simulink model "PREPROCESS"  (R2020b)
settings: Solver=FixedStepAuto  StartTime=0.0  StopTime=31622400  FixedStep=60  RelTol=1e-3
libraries: simulink x30
(part 2 of 2)

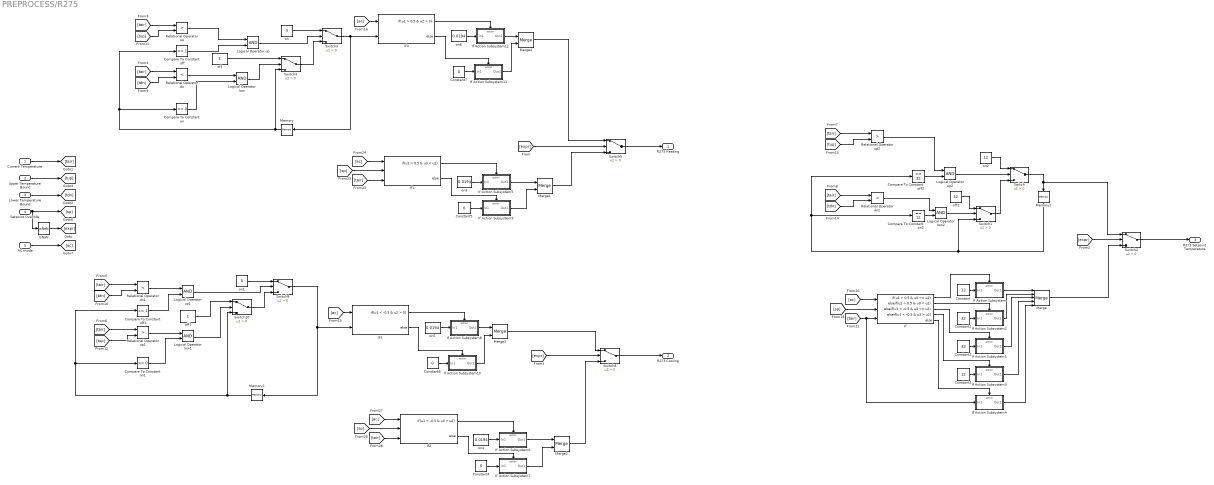
== system PREPROCESS/R275 ==
  Current Temperature : Inport
  Upper Temperature Bound : Inport  Port=2
  Lower Temperature Bound : Inport  Port=3
  Setpoint Override : Inport  Port=4
  AC mode : Inport  Port=5
  Compare To Constant off : simulink/Logic and Bit Operations/Compare To Constant  relop===  const=1  OutDataTypeStr=boolean
  Compare To Constant off1 : simulink/Logic and Bit Operations/Compare To Constant  relop===  const=1  OutDataTypeStr=boolean
  Compare To Constant off2 : simulink/Logic and Bit Operations/Compare To Constant  relop===  const=32  OutDataTypeStr=boolean
  Compare To Constant on : simulink/Logic and Bit Operations/Compare To Constant  relop===  const=0  OutDataTypeStr=boolean
  Compare To Constant on1 : simulink/Logic and Bit Operations/Compare To Constant  relop===  const=0  OutDataTypeStr=boolean
  Compare To Constant on2 : simulink/Logic and Bit Operations/Compare To Constant  relop===  const=12  OutDataTypeStr=boolean
  Constant : Constant  Value=12
  Constant1 : Constant  Value=32
  Constant2 : Constant  Value=32
  Constant3 : Constant  Value=12
  Constant{4..7} (4 alike) : Constant  Value=0
  If : If  NumInputs=3  IfExpression=u1 > 0.5 & u3 >= u2  ElseIfExpressions=u1 > 0.5 & u3 < u2, u1 < -0.5 & u3 <= u2, u1 < -0.5 & u3 > u2
  If Action Subsystem : Subsystem  TreatAsAtomicUnit=on
  If Action Subsystem1 : Subsystem  TreatAsAtomicUnit=on
  If Action Subsystem10 : Subsystem  TreatAsAtomicUnit=on
  If Action Subsystem11 : Subsystem  TreatAsAtomicUnit=on
  If Action Subsystem12 : Subsystem  TreatAsAtomicUnit=on
  If Action Subsystem2 : Subsystem  TreatAsAtomicUnit=on
  If Action Subsystem3 : Subsystem  TreatAsAtomicUnit=on
  If Action Subsystem4 : Subsystem  TreatAsAtomicUnit=on
  If Action Subsystem5 : Subsystem  TreatAsAtomicUnit=on
  If Action Subsystem6 : Subsystem  TreatAsAtomicUnit=on
  If Action Subsystem7 : Subsystem  TreatAsAtomicUnit=on
  If Action Subsystem8 : Subsystem  TreatAsAtomicUnit=on
  If Action Subsystem9 : Subsystem  TreatAsAtomicUnit=on
  If1 : If  NumInputs=3  IfExpression=u1 > 0.5 & u3 < u2
  If2 : If  NumInputs=3  IfExpression=u1 < -0.5 & u3 > u2
  If3 : If  NumInputs=2  IfExpression=u1 < -0.5 & u2 > 0
  If4 : If  NumInputs=2  IfExpression=u1 > 0.5 & u2 > 0
  IsNaN : RelationalOperator  Operator=isNaN  OutDataTypeStr=boolean  RndMeth=Simplest
  Logical Operator low : Logic  AllPortsSameDT=off  OutDataTypeStr=boolean
  Logical Operator low1 : Logic  AllPortsSameDT=off  OutDataTypeStr=boolean
  Logical Operator low2 : Logic  AllPortsSameDT=off  OutDataTypeStr=boolean
  Logical Operator up : Logic  AllPortsSameDT=off  OutDataTypeStr=boolean
  Logical Operator up1 : Logic  AllPortsSameDT=off  OutDataTypeStr=boolean
  Logical Operator up2 : Logic  AllPortsSameDT=off  OutDataTypeStr=boolean
  Memory : Memory
  Memory1 : Memory
  Memory2 : Memory  InitialCondition=12
  Merge : Merge  Inputs=5
  Merge{1..4} (4 alike) : Merge
  Relational Operator dn : RelationalOperator  Operator=<  OutDataTypeStr=boolean  RndMeth=Simplest
  Relational Operator dn1 : RelationalOperator  Operator=<  OutDataTypeStr=boolean  RndMeth=Simplest
  Relational Operator dn2 : RelationalOperator  Operator=<  OutDataTypeStr=boolean  RndMeth=Simplest
  Relational Operator up : RelationalOperator  Operator=>  OutDataTypeStr=boolean  RndMeth=Simplest
  Relational Operator up1 : RelationalOperator  Operator=>  OutDataTypeStr=boolean  RndMeth=Simplest
  Relational Operator up2 : RelationalOperator  Operator=>  OutDataTypeStr=boolean  RndMeth=Simplest
  Switch{,1..5,8..10} (9 alike) : Switch  Criteria=u2 > Threshold
  off : Constant
  off1 : Constant
  off2 : Constant  Value=32
  on : Constant  Value=0
  on1 : Constant  Value=0
  on2 : Constant  Value=12
  on{3..6} (4 alike) : Constant  Value=0.0194
  R273 Heating : Outport
  R273 Cooling : Outport  Port=2
  R273 Setpoint Temperature : Outport  Port=3
  wires:
  If3/1 -> If Action Subsystem8/Action
  If2/1 -> If Action Subsystem6/Action
  If Action Subsystem3/1(Out1) -> Merge/4
  [tair] -> If Action Subsystem4/1(In1), If/3
  [sp] -> If/2
  Relational Operator dn/1 -> Logical Operator low/1
  [tup] -> Relational Operator up/2
  Constant7/1 -> If Action Subsystem11/1(In1)
  [expr] -> Switch5/2
  If1/2 -> If Action Subsystem9/Action
  Merge2/1 -> Switch8/3
  on6/1 -> If Action Subsystem12/1(In1)
  If Action Subsystem10/1(Out1) -> Merge3/2
  [tair] -> If1/3
  on2/1 -> Switch/1
  IsNaN/1 -> [expr]
  If4/2 -> If Action Subsystem11/Action
  If Action Subsystem11/1(Out1) -> Merge4/2
  If4/1 -> If Action Subsystem12/Action
  Constant4/1 -> If Action Subsystem7/1(In1)
  Switch8/1 -> R273 Cooling/1
  [sp] -> If1/2
  If Action Subsystem8/1(Out1) -> Merge3/1
  on4/1 -> If Action Subsystem6/1(In1)
  If/5 -> If Action Subsystem4/Action
  [ac] -> If4/1
  Switch4/1 -> Switch3/3
  Switch9/1 -> If3/2, Memory1/1
  [sp] -> If2/2
  If3/2 -> If Action Subsystem10/Action
  Switch5/1 -> R273 Heating/1
  Constant6/1 -> If Action Subsystem10/1(In1)
  Relational Operator up2/1 -> Logical Operator up2/1
  on5/1 -> If Action Subsystem8/1(In1)
  Compare To Constant on/1 -> Logical Operator low/2
  Lower Temperature Bound/1 -> [tdn]
  Constant2/1 -> If Action Subsystem1/1(In1)
  If Action Subsystem4/1(Out1) -> Merge/5
  Compare To Constant off/1 -> Logical Operator up/2
  Merge4/1 -> Switch5/1
  If1/1 -> If Action Subsystem5/Action
  [ac] -> If3/1
  Merge3/1 -> Switch8/1
  AC mode/1 -> [ac]
  Logical Operator up/1 -> Switch3/2
  If Action Subsystem6/1(Out1) -> Merge2/1
  Memory/1 -> Compare To Constant on/1, Compare To Constant off/1, Switch4/3
  If/2 -> If Action Subsystem2/Action
  on3/1 -> If Action Subsystem5/1(In1)
  Merge1/1 -> Switch5/3
  If Action Subsystem9/1(Out1) -> Merge1/2
  If Action Subsystem/1(Out1) -> Merge/1
  Logical Operator low1/1 -> Switch10/2
  If/3 -> If Action Subsystem1/Action
  [tair] -> Relational Operator up2/1
  off1/1 -> Switch10/1
  [ac] -> If2/1
  Setpoint Override/1 -> IsNaN/1, [sp]
  Relational Operator dn2/1 -> Logical Operator low2/1
  If Action Subsystem12/1(Out1) -> Merge4/1
  Compare To Constant off2/1 -> Logical Operator up2/2
  Switch10/1 -> Switch9/3
  [ac] -> If/1
  Relational Operator up1/1 -> Logical Operator low1/1
  Relational Operator dn1/1 -> Logical Operator up1/1
  [tup] -> Relational Operator up1/2
  off/1 -> Switch4/1
  [expr] -> Switch2/2
  [expr] -> Switch8/2
  Constant/1 -> If Action Subsystem/1(In1)
  [tair] -> Relational Operator dn1/1
  [tair] -> Relational Operator up1/1
  [tdn] -> Relational Operator dn2/2
  Constant5/1 -> If Action Subsystem9/1(In1)
  If Action Subsystem7/1(Out1) -> Merge2/2
  Logical Operator low2/1 -> Switch1/2
  [tup] -> Relational Operator up2/2
  Merge/1 -> Switch2/3
  on/1 -> Switch3/1
  Constant3/1 -> If Action Subsystem3/1(In1)
  If/4 -> If Action Subsystem3/Action
  Logical Operator low/1 -> Switch4/2
  [tdn] -> Relational Operator dn1/2
  on1/1 -> Switch9/1
  Logical Operator up1/1 -> Switch9/2
  Compare To Constant off1/1 -> Logical Operator up1/2
  Relational Operator up/1 -> Logical Operator up/1
  Logical Operator up2/1 -> Switch/2
  Current Temperature/1 -> [tair]
  [tair] -> Relational Operator up/1
  [tair] -> Relational Operator dn/1
  If Action Subsystem1/1(Out1) -> Merge/3
  Compare To Constant on2/1 -> Logical Operator low2/2
  [tair] -> If2/3
  Switch3/1 -> Memory/1, If4/2
  Switch/1 -> Switch2/1, Memory2/1
  Constant1/1 -> If Action Subsystem2/1(In1)
  If Action Subsystem5/1(Out1) -> Merge1/1
  [tdn] -> Relational Operator dn/2
  Switch1/1 -> Switch/3
  off2/1 -> Switch1/1
  Memory1/1 -> Compare To Constant on1/1, Compare To Constant off1/1, Switch10/3
  Memory2/1 -> Compare To Constant on2/1, Compare To Constant off2/1, Switch1/3
  Upper Temperature Bound/1 -> [tup]
  Compare To Constant on1/1 -> Logical Operator low1/2
  [tair] -> Relational Operator dn2/1
  If/1 -> If Action Subsystem/Action
  [ac] -> If1/1
  If Action Subsystem2/1(Out1) -> Merge/2
  If2/2 -> If Action Subsystem7/Action
  Switch2/1 -> R273 Setpoint Temperature/1

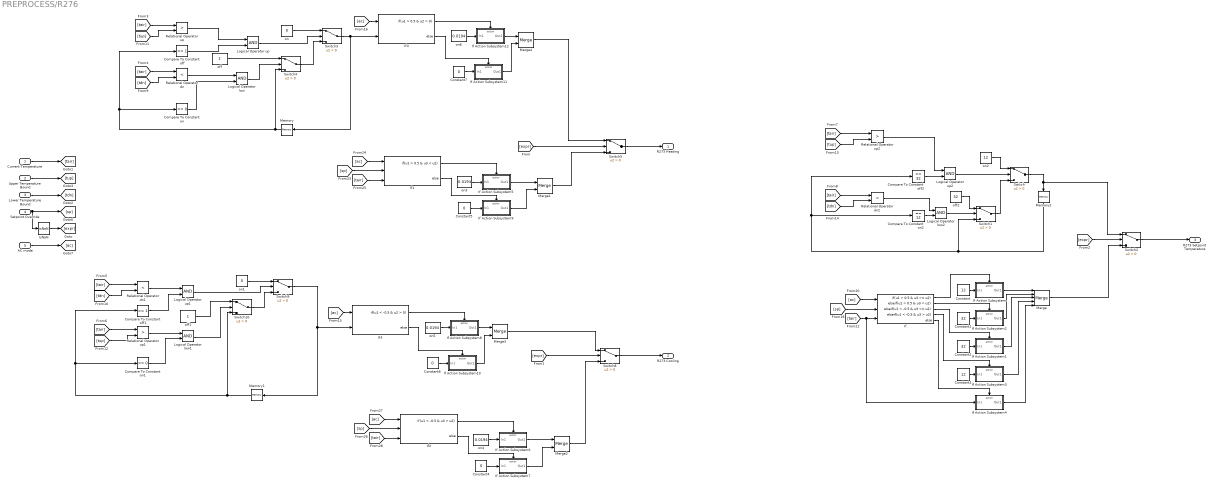
== system PREPROCESS/R276 ==
  Current Temperature : Inport
  Upper Temperature Bound : Inport  Port=2
  Lower Temperature Bound : Inport  Port=3
  Setpoint Override : Inport  Port=4
  AC mode : Inport  Port=5
  Compare To Constant off : simulink/Logic and Bit Operations/Compare To Constant  relop===  const=1  OutDataTypeStr=boolean
  Compare To Constant off1 : simulink/Logic and Bit Operations/Compare To Constant  relop===  const=1  OutDataTypeStr=boolean
  Compare To Constant off2 : simulink/Logic and Bit Operations/Compare To Constant  relop===  const=32  OutDataTypeStr=boolean
  Compare To Constant on : simulink/Logic and Bit Operations/Compare To Constant  relop===  const=0  OutDataTypeStr=boolean
  Compare To Constant on1 : simulink/Logic and Bit Operations/Compare To Constant  relop===  const=0  OutDataTypeStr=boolean
  Compare To Constant on2 : simulink/Logic and Bit Operations/Compare To Constant  relop===  const=12  OutDataTypeStr=boolean
  Constant : Constant  Value=12
  Constant1 : Constant  Value=32
  Constant2 : Constant  Value=32
  Constant3 : Constant  Value=12
  Constant{4..7} (4 alike) : Constant  Value=0
  If : If  NumInputs=3  IfExpression=u1 > 0.5 & u3 >= u2  ElseIfExpressions=u1 > 0.5 & u3 < u2, u1 < -0.5 & u3 <= u2, u1 < -0.5 & u3 > u2
  If Action Subsystem : Subsystem  TreatAsAtomicUnit=on
  If Action Subsystem1 : Subsystem  TreatAsAtomicUnit=on
  If Action Subsystem10 : Subsystem  TreatAsAtomicUnit=on
  If Action Subsystem11 : Subsystem  TreatAsAtomicUnit=on
  If Action Subsystem12 : Subsystem  TreatAsAtomicUnit=on
  If Action Subsystem2 : Subsystem  TreatAsAtomicUnit=on
  If Action Subsystem3 : Subsystem  TreatAsAtomicUnit=on
  If Action Subsystem4 : Subsystem  TreatAsAtomicUnit=on
  If Action Subsystem5 : Subsystem  TreatAsAtomicUnit=on
  If Action Subsystem6 : Subsystem  TreatAsAtomicUnit=on
  If Action Subsystem7 : Subsystem  TreatAsAtomicUnit=on
  If Action Subsystem8 : Subsystem  TreatAsAtomicUnit=on
  If Action Subsystem9 : Subsystem  TreatAsAtomicUnit=on
  If1 : If  NumInputs=3  IfExpression=u1 > 0.5 & u3 < u2
  If2 : If  NumInputs=3  IfExpression=u1 < -0.5 & u3 > u2
  If3 : If  NumInputs=2  IfExpression=u1 < -0.5 & u2 > 0
  If4 : If  NumInputs=2  IfExpression=u1 > 0.5 & u2 > 0
  IsNaN : RelationalOperator  Operator=isNaN  OutDataTypeStr=boolean  RndMeth=Simplest
  Logical Operator low : Logic  AllPortsSameDT=off  OutDataTypeStr=boolean
  Logical Operator low1 : Logic  AllPortsSameDT=off  OutDataTypeStr=boolean
  Logical Operator low2 : Logic  AllPortsSameDT=off  OutDataTypeStr=boolean
  Logical Operator up : Logic  AllPortsSameDT=off  OutDataTypeStr=boolean
  Logical Operator up1 : Logic  AllPortsSameDT=off  OutDataTypeStr=boolean
  Logical Operator up2 : Logic  AllPortsSameDT=off  OutDataTypeStr=boolean
  Memory : Memory
  Memory1 : Memory
  Memory2 : Memory  InitialCondition=12
  Merge : Merge  Inputs=5
  Merge{1..4} (4 alike) : Merge
  Relational Operator dn : RelationalOperator  Operator=<  OutDataTypeStr=boolean  RndMeth=Simplest
  Relational Operator dn1 : RelationalOperator  Operator=<  OutDataTypeStr=boolean  RndMeth=Simplest
  Relational Operator dn2 : RelationalOperator  Operator=<  OutDataTypeStr=boolean  RndMeth=Simplest
  Relational Operator up : RelationalOperator  Operator=>  OutDataTypeStr=boolean  RndMeth=Simplest
  Relational Operator up1 : RelationalOperator  Operator=>  OutDataTypeStr=boolean  RndMeth=Simplest
  Relational Operator up2 : RelationalOperator  Operator=>  OutDataTypeStr=boolean  RndMeth=Simplest
  Switch{,1..5,8..10} (9 alike) : Switch  Criteria=u2 > Threshold
  off : Constant
  off1 : Constant
  off2 : Constant  Value=32
  on : Constant  Value=0
  on1 : Constant  Value=0
  on2 : Constant  Value=12
  on{3..6} (4 alike) : Constant  Value=0.0194
  R273 Heating : Outport
  R273 Cooling : Outport  Port=2
  R273 Setpoint Temperature : Outport  Port=3
  wires:
  Logical Operator low/1 -> Switch4/2
  If/4 -> If Action Subsystem3/Action
  Constant3/1 -> If Action Subsystem3/1(In1)
  Merge/1 -> Switch2/3
  [tup] -> Relational Operator up2/2
  Logical Operator low2/1 -> Switch1/2
  If Action Subsystem9/1(Out1) -> Merge1/2
  Merge1/1 -> Switch5/3
  on3/1 -> If Action Subsystem5/1(In1)
  If Action Subsystem/1(Out1) -> Merge/1
  off/1 -> Switch4/1
  [tair] -> Relational Operator dn1/1
  Relational Operator up1/1 -> Logical Operator low1/1
  [ac] -> If1/1
  Compare To Constant on1/1 -> Logical Operator low1/2
  If/1 -> If Action Subsystem/Action
  Upper Temperature Bound/1 -> [tup]
  [tair] -> Relational Operator dn2/1
  Switch1/1 -> Switch/3
  Memory1/1 -> Compare To Constant on1/1, Compare To Constant off1/1, Switch10/3
  off2/1 -> Switch1/1
  Switch3/1 -> Memory/1, If4/2
  Compare To Constant on2/1 -> Logical Operator low2/2
  Constant1/1 -> If Action Subsystem2/1(In1)
  Switch/1 -> Switch2/1, Memory2/1
  [tair] -> If2/3
  If Action Subsystem1/1(Out1) -> Merge/3
  Switch2/1 -> R273 Setpoint Temperature/1
  If2/2 -> If Action Subsystem7/Action
  If Action Subsystem2/1(Out1) -> Merge/2
  on1/1 -> Switch9/1
  Logical Operator up1/1 -> Switch9/2
  Logical Operator low1/1 -> Switch10/2
  Relational Operator up/1 -> Logical Operator up/1
  [tair] -> Relational Operator up1/1
  [tdn] -> Relational Operator dn2/2
  off1/1 -> Switch10/1
  Constant5/1 -> If Action Subsystem9/1(In1)
  Switch10/1 -> Switch9/3
  Compare To Constant off2/1 -> Logical Operator up2/2
  If/3 -> If Action Subsystem1/Action
  If Action Subsystem3/1(Out1) -> Merge/4
  If2/1 -> If Action Subsystem6/Action
  Memory/1 -> Compare To Constant on/1, Compare To Constant off/1, Switch4/3
  [tdn] -> Relational Operator dn/2
  AC mode/1 -> [ac]
  [ac] -> If3/1
  Compare To Constant off/1 -> Logical Operator up/2
  Constant2/1 -> If Action Subsystem1/1(In1)
  If Action Subsystem4/1(Out1) -> Merge/5
  on5/1 -> If Action Subsystem8/1(In1)
  Logical Operator up/1 -> Switch3/2
  If Action Subsystem7/1(Out1) -> Merge2/2
  Constant6/1 -> If Action Subsystem10/1(In1)
  Relational Operator up2/1 -> Logical Operator up2/1
  Switch5/1 -> R273 Heating/1
  If Action Subsystem5/1(Out1) -> Merge1/1
  If3/2 -> If Action Subsystem10/Action
  If1/1 -> If Action Subsystem5/Action
  Switch4/1 -> Switch3/3
  If/5 -> If Action Subsystem4/Action
  [ac] -> If4/1
  on4/1 -> If Action Subsystem6/1(In1)
  Lower Temperature Bound/1 -> [tdn]
  If Action Subsystem8/1(Out1) -> Merge3/1
  Merge4/1 -> Switch5/1
  Switch8/1 -> R273 Cooling/1
  If4/1 -> If Action Subsystem12/Action
  If Action Subsystem11/1(Out1) -> Merge4/2
  [tair] -> If1/3
  If4/2 -> If Action Subsystem11/Action
  Memory2/1 -> Compare To Constant on2/1, Compare To Constant off2/1, Switch1/3
  IsNaN/1 -> [expr]
  on2/1 -> Switch/1
  If3/1 -> If Action Subsystem8/Action
  Constant7/1 -> If Action Subsystem11/1(In1)
  If1/2 -> If Action Subsystem9/Action
  Merge2/1 -> Switch8/3
  [expr] -> Switch5/2
  on6/1 -> If Action Subsystem12/1(In1)
  [tup] -> Relational Operator up/2
  Relational Operator dn/1 -> Logical Operator low/1
  Compare To Constant on/1 -> Logical Operator low/2
  Merge3/1 -> Switch8/1
  on/1 -> Switch3/1
  [tair] -> If Action Subsystem4/1(In1), If/3
  Constant/1 -> If Action Subsystem/1(In1)
  [expr] -> Switch2/2
  [sp] -> If2/2
  [expr] -> Switch8/2
  [ac] -> If2/1
  [tup] -> Relational Operator up1/2
  Relational Operator dn1/1 -> Logical Operator up1/1
  Compare To Constant off1/1 -> Logical Operator up1/2
  If Action Subsystem6/1(Out1) -> Merge2/1
  Logical Operator up2/1 -> Switch/2
  Relational Operator dn2/1 -> Logical Operator low2/1
  Constant4/1 -> If Action Subsystem7/1(In1)
  [tdn] -> Relational Operator dn1/2
  [sp] -> If1/2
  Current Temperature/1 -> [tair]
  If/2 -> If Action Subsystem2/Action
  If Action Subsystem12/1(Out1) -> Merge4/1
  [sp] -> If/2
  [tair] -> Relational Operator up/1
  [ac] -> If/1
  Setpoint Override/1 -> IsNaN/1, [sp]
  [tair] -> Relational Operator up2/1
  Switch9/1 -> If3/2, Memory1/1
  If Action Subsystem10/1(Out1) -> Merge3/2
  [tair] -> Relational Operator dn/1

== system PREPROCESS/Subsystem ==
  In1 : Inport
  In2 : Inport  Port=2
  IsNaN2 : RelationalOperator  Operator=isNaN  OutDataTypeStr=boolean  RndMeth=Simplest
  Saturation2 : Saturate  UpperLimit=1000  LowerLimit=0
  Switch3 : Switch  Criteria=u2 > Threshold
  Out1 : Outport
  wires:
  In2/1 -> IsNaN2/1, Switch3/3
  Switch3/1 -> Saturation2/1
  IsNaN2/1 -> Switch3/2
  In1/1 -> Switch3/1
  Saturation2/1 -> Out1/1

== system PREPROCESS/Subsystem1 ==
  In1 : Inport
  In2 : Inport  Port=2
  IsNaN1 : RelationalOperator  Operator=isNaN  OutDataTypeStr=boolean  RndMeth=Simplest
  Saturation1 : Saturate  UpperLimit=5000  LowerLimit=0
  Switch2 : Switch  Criteria=u2 > Threshold
  Out1 : Outport
  wires:
  Saturation1/1 -> Out1/1
  In2/1 -> Switch2/3, IsNaN1/1
  IsNaN1/1 -> Switch2/2
  Switch2/1 -> Saturation1/1
  In1/1 -> Switch2/1

== system PREPROCESS/Subsystem2 ==
  In1 : Inport
  In2 : Inport  Port=2
  IsNaN : RelationalOperator  Operator=isNaN  OutDataTypeStr=boolean  RndMeth=Simplest
  Saturation : Saturate  UpperLimit=1000  LowerLimit=0
  Switch1 : Switch  Criteria=u2 > Threshold
  Out1 : Outport
  wires:
  IsNaN/1 -> Switch1/2
  In2/1 -> Switch1/3, IsNaN/1
  Switch1/1 -> Saturation/1
  In1/1 -> Switch1/1
  Saturation/1 -> Out1/1

== system PREPROCESS/R272/If Action Subsystem ==
  In1 : Inport
  Action Port : ActionPort  ActionPortLabel=if(u1 > 0.5 & u3 >= u2)
  Out1 : Outport
  wires:
  In1/1 -> Out1/1

== system PREPROCESS/R272/If Action Subsystem1 ==
  In1 : Inport
  Action Port : ActionPort  ActionPortLabel=elseif( u1 < -0.5 & u3 <= u2)
  Out1 : Outport
  wires:
  In1/1 -> Out1/1

== system PREPROCESS/R272/If Action Subsystem10 ==
  In1 : Inport
  Action Port : ActionPort  ActionPortLabel=else
  Out1 : Outport
  wires:
  In1/1 -> Out1/1

== system PREPROCESS/R272/If Action Subsystem11 ==
  In1 : Inport
  Action Port : ActionPort  ActionPortLabel=else
  Out1 : Outport
  wires:
  In1/1 -> Out1/1

== system PREPROCESS/R272/If Action Subsystem12 ==
  In1 : Inport
  Action Port : ActionPort  ActionPortLabel=if(u1 > 0.5 & u2 > 0)
  Out1 : Outport
  wires:
  In1/1 -> Out1/1

== system PREPROCESS/R272/If Action Subsystem2 ==
  In1 : Inport
  Action Port : ActionPort  ActionPortLabel=elseif(u1 > 0.5 & u3 < u2)
  Out1 : Outport
  wires:
  In1/1 -> Out1/1

== system PREPROCESS/R272/If Action Subsystem3 ==
  In1 : Inport
  Action Port : ActionPort  ActionPortLabel=elseif( u1 < -0.5 & u3 > u2)
  Out1 : Outport
  wires:
  In1/1 -> Out1/1

== system PREPROCESS/R272/If Action Subsystem4 ==
  In1 : Inport
  Action Port : ActionPort  ActionPortLabel=else
  Out1 : Outport
  wires:
  In1/1 -> Out1/1

== system PREPROCESS/R272/If Action Subsystem5 ==
  In1 : Inport
  Action Port : ActionPort  ActionPortLabel=if(u1 > 0.5 & u3 < u2)
  Out1 : Outport
  wires:
  In1/1 -> Out1/1

== system PREPROCESS/R272/If Action Subsystem6 ==
  In1 : Inport
  Action Port : ActionPort  ActionPortLabel=if(u1 < -0.5 & u3 > u2)
  Out1 : Outport
  wires:
  In1/1 -> Out1/1

== system PREPROCESS/R272/If Action Subsystem7 ==
  In1 : Inport
  Action Port : ActionPort  ActionPortLabel=else
  Out1 : Outport
  wires:
  In1/1 -> Out1/1

== system PREPROCESS/R272/If Action Subsystem8 ==
  In1 : Inport
  Action Port : ActionPort  ActionPortLabel=if(u1 < -0.5 & u2 > 0)
  Out1 : Outport
  wires:
  In1/1 -> Out1/1

== system PREPROCESS/R272/If Action Subsystem9 ==
  In1 : Inport
  Action Port : ActionPort  ActionPortLabel=else
  Out1 : Outport
  wires:
  In1/1 -> Out1/1

== system PREPROCESS/R273/If Action Subsystem ==
  In1 : Inport
  Action Port : ActionPort  ActionPortLabel=if(u1 > 0.5 & u3 >= u2)
  Out1 : Outport
  wires:
  In1/1 -> Out1/1

== system PREPROCESS/R273/If Action Subsystem1 ==
  In1 : Inport
  Action Port : ActionPort  ActionPortLabel=elseif( u1 < -0.5 & u3 <= u2)
  Out1 : Outport
  wires:
  In1/1 -> Out1/1

== system PREPROCESS/R273/If Action Subsystem10 ==
  In1 : Inport
  Action Port : ActionPort  ActionPortLabel=else
  Out1 : Outport
  wires:
  In1/1 -> Out1/1

== system PREPROCESS/R273/If Action Subsystem11 ==
  In1 : Inport
  Action Port : ActionPort  ActionPortLabel=else
  Out1 : Outport
  wires:
  In1/1 -> Out1/1

== system PREPROCESS/R273/If Action Subsystem12 ==
  In1 : Inport
  Action Port : ActionPort  ActionPortLabel=if(u1 > 0.5 & u2 > 0)
  Out1 : Outport
  wires:
  In1/1 -> Out1/1

== system PREPROCESS/R273/If Action Subsystem2 ==
  In1 : Inport
  Action Port : ActionPort  ActionPortLabel=elseif(u1 > 0.5 & u3 < u2)
  Out1 : Outport
  wires:
  In1/1 -> Out1/1

== system PREPROCESS/R273/If Action Subsystem3 ==
  In1 : Inport
  Action Port : ActionPort  ActionPortLabel=elseif( u1 < -0.5 & u3 > u2)
  Out1 : Outport
  wires:
  In1/1 -> Out1/1

== system PREPROCESS/R273/If Action Subsystem4 ==
  In1 : Inport
  Action Port : ActionPort  ActionPortLabel=else
  Out1 : Outport
  wires:
  In1/1 -> Out1/1

== system PREPROCESS/R273/If Action Subsystem5 ==
  In1 : Inport
  Action Port : ActionPort  ActionPortLabel=if(u1 > 0.5 & u3 < u2)
  Out1 : Outport
  wires:
  In1/1 -> Out1/1

== system PREPROCESS/R273/If Action Subsystem6 ==
  In1 : Inport
  Action Port : ActionPort  ActionPortLabel=if(u1 < -0.5 & u3 > u2)
  Out1 : Outport
  wires:
  In1/1 -> Out1/1

== system PREPROCESS/R273/If Action Subsystem7 ==
  In1 : Inport
  Action Port : ActionPort  ActionPortLabel=else
  Out1 : Outport
  wires:
  In1/1 -> Out1/1

== system PREPROCESS/R273/If Action Subsystem8 ==
  In1 : Inport
  Action Port : ActionPort  ActionPortLabel=if(u1 < -0.5 & u2 > 0)
  Out1 : Outport
  wires:
  In1/1 -> Out1/1

== system PREPROCESS/R273/If Action Subsystem9 ==
  In1 : Inport
  Action Port : ActionPort  ActionPortLabel=else
  Out1 : Outport
  wires:
  In1/1 -> Out1/1

== system PREPROCESS/R274/If Action Subsystem ==
  In1 : Inport
  Action Port : ActionPort  ActionPortLabel=if(u1 > 0.5 & u3 >= u2)
  Out1 : Outport
  wires:
  In1/1 -> Out1/1

== system PREPROCESS/R274/If Action Subsystem1 ==
  In1 : Inport
  Action Port : ActionPort  ActionPortLabel=elseif( u1 < -0.5 & u3 <= u2)
  Out1 : Outport
  wires:
  In1/1 -> Out1/1

== system PREPROCESS/R274/If Action Subsystem10 ==
  In1 : Inport
  Action Port : ActionPort  ActionPortLabel=else
  Out1 : Outport
  wires:
  In1/1 -> Out1/1

== system PREPROCESS/R274/If Action Subsystem11 ==
  In1 : Inport
  Action Port : ActionPort  ActionPortLabel=else
  Out1 : Outport
  wires:
  In1/1 -> Out1/1

== system PREPROCESS/R274/If Action Subsystem12 ==
  In1 : Inport
  Action Port : ActionPort  ActionPortLabel=if(u1 > 0.5 & u2 > 0)
  Out1 : Outport
  wires:
  In1/1 -> Out1/1

== system PREPROCESS/R274/If Action Subsystem2 ==
  In1 : Inport
  Action Port : ActionPort  ActionPortLabel=elseif(u1 > 0.5 & u3 < u2)
  Out1 : Outport
  wires:
  In1/1 -> Out1/1

== system PREPROCESS/R274/If Action Subsystem3 ==
  In1 : Inport
  Action Port : ActionPort  ActionPortLabel=elseif( u1 < -0.5 & u3 > u2)
  Out1 : Outport
  wires:
  In1/1 -> Out1/1

== system PREPROCESS/R274/If Action Subsystem4 ==
  In1 : Inport
  Action Port : ActionPort  ActionPortLabel=else
  Out1 : Outport
  wires:
  In1/1 -> Out1/1

== system PREPROCESS/R274/If Action Subsystem5 ==
  In1 : Inport
  Action Port : ActionPort  ActionPortLabel=if(u1 > 0.5 & u3 < u2)
  Out1 : Outport
  wires:
  In1/1 -> Out1/1

== system PREPROCESS/R274/If Action Subsystem6 ==
  In1 : Inport
  Action Port : ActionPort  ActionPortLabel=if(u1 < -0.5 & u3 > u2)
  Out1 : Outport
  wires:
  In1/1 -> Out1/1

== system PREPROCESS/R274/If Action Subsystem7 ==
  In1 : Inport
  Action Port : ActionPort  ActionPortLabel=else
  Out1 : Outport
  wires:
  In1/1 -> Out1/1

== system PREPROCESS/R274/If Action Subsystem8 ==
  In1 : Inport
  Action Port : ActionPort  ActionPortLabel=if(u1 < -0.5 & u2 > 0)
  Out1 : Outport
  wires:
  In1/1 -> Out1/1

== system PREPROCESS/R274/If Action Subsystem9 ==
  In1 : Inport
  Action Port : ActionPort  ActionPortLabel=else
  Out1 : Outport
  wires:
  In1/1 -> Out1/1

== system PREPROCESS/R275/If Action Subsystem ==
  In1 : Inport
  Action Port : ActionPort  ActionPortLabel=if(u1 > 0.5 & u3 >= u2)
  Out1 : Outport
  wires:
  In1/1 -> Out1/1

== system PREPROCESS/R275/If Action Subsystem1 ==
  In1 : Inport
  Action Port : ActionPort  ActionPortLabel=elseif( u1 < -0.5 & u3 <= u2)
  Out1 : Outport
  wires:
  In1/1 -> Out1/1

== system PREPROCESS/R275/If Action Subsystem10 ==
  In1 : Inport
  Action Port : ActionPort  ActionPortLabel=else
  Out1 : Outport
  wires:
  In1/1 -> Out1/1

== system PREPROCESS/R275/If Action Subsystem11 ==
  In1 : Inport
  Action Port : ActionPort  ActionPortLabel=else
  Out1 : Outport
  wires:
  In1/1 -> Out1/1

== system PREPROCESS/R275/If Action Subsystem12 ==
  In1 : Inport
  Action Port : ActionPort  ActionPortLabel=if(u1 > 0.5 & u2 > 0)
  Out1 : Outport
  wires:
  In1/1 -> Out1/1

== system PREPROCESS/R275/If Action Subsystem2 ==
  In1 : Inport
  Action Port : ActionPort  ActionPortLabel=elseif(u1 > 0.5 & u3 < u2)
  Out1 : Outport
  wires:
  In1/1 -> Out1/1

== system PREPROCESS/R275/If Action Subsystem3 ==
  In1 : Inport
  Action Port : ActionPort  ActionPortLabel=elseif( u1 < -0.5 & u3 > u2)
  Out1 : Outport
  wires:
  In1/1 -> Out1/1

== system PREPROCESS/R275/If Action Subsystem4 ==
  In1 : Inport
  Action Port : ActionPort  ActionPortLabel=else
  Out1 : Outport
  wires:
  In1/1 -> Out1/1

== system PREPROCESS/R275/If Action Subsystem5 ==
  In1 : Inport
  Action Port : ActionPort  ActionPortLabel=if(u1 > 0.5 & u3 < u2)
  Out1 : Outport
  wires:
  In1/1 -> Out1/1

== system PREPROCESS/R275/If Action Subsystem6 ==
  In1 : Inport
  Action Port : ActionPort  ActionPortLabel=if(u1 < -0.5 & u3 > u2)
  Out1 : Outport
  wires:
  In1/1 -> Out1/1

== system PREPROCESS/R275/If Action Subsystem7 ==
  In1 : Inport
  Action Port : ActionPort  ActionPortLabel=else
  Out1 : Outport
  wires:
  In1/1 -> Out1/1

== system PREPROCESS/R275/If Action Subsystem8 ==
  In1 : Inport
  Action Port : ActionPort  ActionPortLabel=if(u1 < -0.5 & u2 > 0)
  Out1 : Outport
  wires:
  In1/1 -> Out1/1

== system PREPROCESS/R275/If Action Subsystem9 ==
  In1 : Inport
  Action Port : ActionPort  ActionPortLabel=else
  Out1 : Outport
  wires:
  In1/1 -> Out1/1

== system PREPROCESS/R276/If Action Subsystem ==
  In1 : Inport
  Action Port : ActionPort  ActionPortLabel=if(u1 > 0.5 & u3 >= u2)
  Out1 : Outport
  wires:
  In1/1 -> Out1/1

== system PREPROCESS/R276/If Action Subsystem1 ==
  In1 : Inport
  Action Port : ActionPort  ActionPortLabel=elseif( u1 < -0.5 & u3 <= u2)
  Out1 : Outport
  wires:
  In1/1 -> Out1/1

== system PREPROCESS/R276/If Action Subsystem10 ==
  In1 : Inport
  Action Port : ActionPort  ActionPortLabel=else
  Out1 : Outport
  wires:
  In1/1 -> Out1/1

== system PREPROCESS/R276/If Action Subsystem11 ==
  In1 : Inport
  Action Port : ActionPort  ActionPortLabel=else
  Out1 : Outport
  wires:
  In1/1 -> Out1/1

== system PREPROCESS/R276/If Action Subsystem12 ==
  In1 : Inport
  Action Port : ActionPort  ActionPortLabel=if(u1 > 0.5 & u2 > 0)
  Out1 : Outport
  wires:
  In1/1 -> Out1/1

== system PREPROCESS/R276/If Action Subsystem2 ==
  In1 : Inport
  Action Port : ActionPort  ActionPortLabel=elseif(u1 > 0.5 & u3 < u2)
  Out1 : Outport
  wires:
  In1/1 -> Out1/1

== system PREPROCESS/R276/If Action Subsystem3 ==
  In1 : Inport
  Action Port : ActionPort  ActionPortLabel=elseif( u1 < -0.5 & u3 > u2)
  Out1 : Outport
  wires:
  In1/1 -> Out1/1

== system PREPROCESS/R276/If Action Subsystem4 ==
  In1 : Inport
  Action Port : ActionPort  ActionPortLabel=else
  Out1 : Outport
  wires:
  In1/1 -> Out1/1

== system PREPROCESS/R276/If Action Subsystem5 ==
  In1 : Inport
  Action Port : ActionPort  ActionPortLabel=if(u1 > 0.5 & u3 < u2)
  Out1 : Outport
  wires:
  In1/1 -> Out1/1

== system PREPROCESS/R276/If Action Subsystem6 ==
  In1 : Inport
  Action Port : ActionPort  ActionPortLabel=if(u1 < -0.5 & u3 > u2)
  Out1 : Outport
  wires:
  In1/1 -> Out1/1

== system PREPROCESS/R276/If Action Subsystem7 ==
  In1 : Inport
  Action Port : ActionPort  ActionPortLabel=else
  Out1 : Outport
  wires:
  In1/1 -> Out1/1

== system PREPROCESS/R276/If Action Subsystem8 ==
  In1 : Inport
  Action Port : ActionPort  ActionPortLabel=if(u1 < -0.5 & u2 > 0)
  Out1 : Outport
  wires:
  In1/1 -> Out1/1

== system PREPROCESS/R276/If Action Subsystem9 ==
  In1 : Inport
  Action Port : ActionPort  ActionPortLabel=else
  Out1 : Outport
  wires:
  In1/1 -> Out1/1
